simulink model "WW_ST_ESP_ESM_2016a"  (R2017b)
settings: Solver=ode1  StartTime=0.0  StopTime=SIM_time  FixedStep=stepsize  RelTol=1e-3  EnableMultiTasking=on
values from neighbouring files (symbols this model uses):
  A = 2.26    [ST_einspur_parameter.m]
  brems_k_max = 25000    [ST_einspur_parameter.m]
  cw = 0.32    [ST_einspur_parameter.m]
  delta_lr = 0    [ST_einspur_parameter_dynamik.m]    (also in ST_einspur_parameter_sinus.m = 90; ST_einspur_parameter_sprung.m = 90)
  fah_dkv = 0.6    [ST_einspur_parameter_dynamik.m]    (also in ST_einspur_parameter_sinus.m = 0.2; ST_einspur_parameter_sprung.m)
  fzg_Jz = 3489    [ST_einspur_parameter.m]
  fzg_l = 2.758    [ST_einspur_parameter.m]
  fzg_lh = fzg_l-fzg_lv    (= 1.158)    [ST_einspur_parameter.m]
  fzg_lv = 1.6    [ST_einspur_parameter.m]
  fzg_m = 1700    [ST_einspur_parameter.m]
  fzg_s = 1.7    [ST_einspur_parameter.m]
  g = 9.81    [ST_einspur_parameter.m]
  h_sp = 0.56    [ST_einspur_parameter.m]
  i_diff = 3.5    [ST_einspur_parameter.m]
  i_getr = 4.2    [ST_einspur_parameter.m]
  i_lenk = 18    [ST_einspur_parameter.m]
  init_v0 = 5/3.6    (= 1.38888888889)    [ST_einspur_parameter_dynamik.m]    (also in ST_einspur_parameter_sinus.m = 13.8888888889; ST_einspur_parameter_sprung.m = 11.1111111111)
  len_wahl = 1    [ST_einspur_parameter_dynamik.m]    (also in ST_einspur_parameter_sinus.m = 2; ST_einspur_parameter_sprung.m = 3)
  mue_h = 1.0    (= 1)    [ST_einspur_parameter.m]
  mue_v = 1.0    (= 1)    [ST_einspur_parameter.m]
  omega_max = 630    [ST_einspur_parameter.m]
  p_max = 110000    [ST_einspur_parameter.m]
  rad_r = 0.31    [ST_einspur_parameter.m]
  rho = 1.226    [ST_einspur_parameter.m]
  sin_freq = pi/2    (= 1.57079632679)    [ST_einspur_parameter_dynamik.m]    (also in ST_einspur_parameter_sinus.m = 1.0471975512; ST_einspur_parameter_sprung.m)
  step_time = 1    [ST_einspur_parameter_dynamik.m]    (also in ST_einspur_parameter_sinus.m; ST_einspur_parameter_sprung.m = 3)
  sw_ESP = 1    [ST_einspur_parameter_sinus.m]    (also in ST_einspur_parameter_sprung.m)
libraries: simulink x2
(part 2 of 2)

== system WW_ST_ESP_ESM_2016a/Regelsysteme/ESP/Sensorik/Gierratensensor ==
  psi_p : Inport
  Offset : Constant  Value=0.01
  Product : Product  RndMeth=Zero
  Rate Transition : RateTransition
  Rauschamplitude : Constant  Value=0.004
  Sum : Sum  Inputs=+++
  Uniform Random Number : UniformRandomNumber  SampleTime=0.1
  psi_p_mess : Outport
  wires:
  psi_p/1 -> Sum/1
  Product/1 -> Sum/2
  Rauschamplitude/1 -> Product/1
  Rate Transition/1 -> Product/2
  Offset/1 -> Sum/3
  Sum/1 -> psi_p_mess/1
  Uniform Random Number/1 -> Rate Transition/1

== system WW_ST_ESP_ESM_2016a/Regelsysteme/ESP/Sensorik/Schwimmwinkelsensor ==
  beta : Inport
  Offset : Constant  Value=0.01
  Product : Product  RndMeth=Zero
  Rate Transition : RateTransition
  Rauschamplitude : Constant  Value=0.01
  Sum : Sum  Inputs=+++
  Uniform Random Number : UniformRandomNumber  SampleTime=0.1
  beta_mess : Outport
  wires:
  beta/1 -> Sum/1
  Product/1 -> Sum/2
  Rauschamplitude/1 -> Product/1
  Rate Transition/1 -> Product/2
  Offset/1 -> Sum/3
  Sum/1 -> beta_mess/1
  Uniform Random Number/1 -> Rate Transition/1

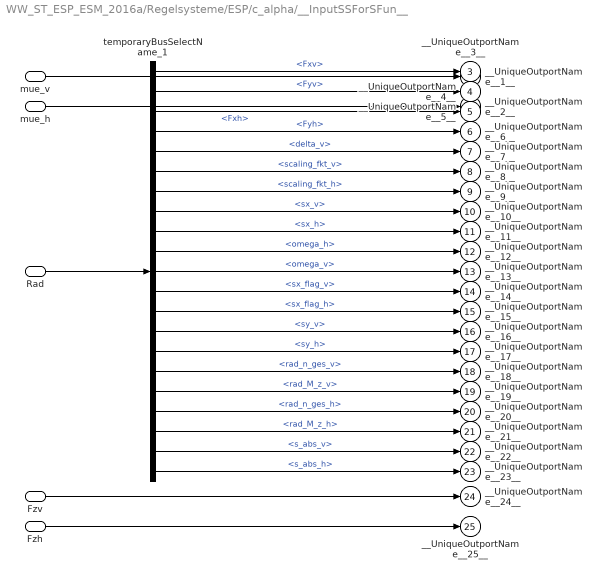
== system WW_ST_ESP_ESM_2016a/Regelsysteme/ESP/c_alpha/__InputSSForSFun__ ==
  mue_v : Inport
  mue_h : Inport  Port=2
  Rad : Inport  Port=3
  Fzv : Inport  Port=4
  Fzh : Inport  Port=5
  temporaryBusSelectName_1 : BusSelector  OutputSignals=Fxv,Fyv,Fxh,Fyh,delta_v,scaling_fkt_v,scaling_fkt_h,sx_v,sx_h,omega_h,omega_v,sx_flag_v,sx_flag_h,sy_v,sy_h,rad_Mz.rad_n_ges_v,rad_Mz.rad_M_z_v,rad_Mz.rad_n_ges_h,rad_Mz.rad_M_z_h,s_abs_v,s_abs_h
  __UniqueOutportName__1__ : Outport
  __UniqueOutportName__2__ : Outport  Port=2
  __UniqueOutportName__3__ : Outport  Port=3
  __UniqueOutportName__4__ : Outport  Port=4
  __UniqueOutportName__5__ : Outport  Port=5
  __UniqueOutportName__6__ : Outport  Port=6
  __UniqueOutportName__7__ : Outport  Port=7
  __UniqueOutportName__8__ : Outport  Port=8
  __UniqueOutportName__9__ : Outport  Port=9
  __UniqueOutportName__10__ : Outport  Port=10
  __UniqueOutportName__11__ : Outport  Port=11
  __UniqueOutportName__12__ : Outport  Port=12
  __UniqueOutportName__13__ : Outport  Port=13
  __UniqueOutportName__14__ : Outport  Port=14
  __UniqueOutportName__15__ : Outport  Port=15
  __UniqueOutportName__16__ : Outport  Port=16
  __UniqueOutportName__17__ : Outport  Port=17
  __UniqueOutportName__18__ : Outport  Port=18
  __UniqueOutportName__19__ : Outport  Port=19
  __UniqueOutportName__20__ : Outport  Port=20
  __UniqueOutportName__21__ : Outport  Port=21
  __UniqueOutportName__22__ : Outport  Port=22
  __UniqueOutportName__23__ : Outport  Port=23
  __UniqueOutportName__24__ : Outport  Port=24
  __UniqueOutportName__25__ : Outport  Port=25
  wires:
  Fzh/1 -> __UniqueOutportName__25__/1
  Fzv/1 -> __UniqueOutportName__24__/1
  temporaryBusSelectName_1/21 -> __UniqueOutportName__23__/1  "<s_abs_h>"
  temporaryBusSelectName_1/20 -> __UniqueOutportName__22__/1  "<s_abs_v>"
  temporaryBusSelectName_1/19 -> __UniqueOutportName__21__/1  "<rad_M_z_h>"
  temporaryBusSelectName_1/18 -> __UniqueOutportName__20__/1  "<rad_n_ges_h>"
  temporaryBusSelectName_1/17 -> __UniqueOutportName__19__/1  "<rad_M_z_v>"
  temporaryBusSelectName_1/16 -> __UniqueOutportName__18__/1  "<rad_n_ges_v>"
  temporaryBusSelectName_1/15 -> __UniqueOutportName__17__/1  "<sy_h>"
  temporaryBusSelectName_1/14 -> __UniqueOutportName__16__/1  "<sy_v>"
  temporaryBusSelectName_1/13 -> __UniqueOutportName__15__/1  "<sx_flag_h>"
  temporaryBusSelectName_1/12 -> __UniqueOutportName__14__/1  "<sx_flag_v>"
  temporaryBusSelectName_1/11 -> __UniqueOutportName__13__/1  "<omega_v>"
  temporaryBusSelectName_1/10 -> __UniqueOutportName__12__/1  "<omega_h>"
  temporaryBusSelectName_1/9 -> __UniqueOutportName__11__/1  "<sx_h>"
  temporaryBusSelectName_1/8 -> __UniqueOutportName__10__/1  "<sx_v>"
  temporaryBusSelectName_1/7 -> __UniqueOutportName__9__/1  "<scaling_fkt_h>"
  temporaryBusSelectName_1/6 -> __UniqueOutportName__8__/1  "<scaling_fkt_v>"
  temporaryBusSelectName_1/5 -> __UniqueOutportName__7__/1  "<delta_v>"
  temporaryBusSelectName_1/4 -> __UniqueOutportName__6__/1  "<Fyh>"
  temporaryBusSelectName_1/3 -> __UniqueOutportName__5__/1  "<Fxh>"
  temporaryBusSelectName_1/2 -> __UniqueOutportName__4__/1  "<Fyv>"
  temporaryBusSelectName_1/1 -> __UniqueOutportName__3__/1  "<Fxv>"
  mue_h/1 -> __UniqueOutportName__2__/1
  mue_v/1 -> __UniqueOutportName__1__/1
  Rad/1 -> temporaryBusSelectName_1/1

== system WW_ST_ESP_ESM_2016a/Regelsysteme/ESP/c_alpha/__OutputSSForSFun__ ==
  __UniqueInportName__1__ : Inport
  __UniqueInportName__2__ : Inport  Port=2
  c_alpha_v : Outport
  c_alpha_h : Outport  Port=2
  wires:
  __UniqueInportName__2__/1 -> c_alpha_h/1
  __UniqueInportName__1__/1 -> c_alpha_v/1

== matlab function WW_ST_ESP_ESM_2016a/Regelsysteme/ESP/Subsystem/D-Anteil ==
  data: psi_p input; y output; v input
function y = fcn(psi_p,v)

% D-Regelparameter von psi_p
if v>=0 & v<=70;
    Kd_psi_p=(-1/70).*v+1;
else if v>70 & v<=100;
        Kd_psi_p =0;
else 
    Kd_psi_p = nan;
    end
end

Kd = 1;

y = Kd.*(Kd_psi_p .* psi_p); % delta_Mz(D)
end

== matlab function WW_ST_ESP_ESM_2016a/Regelsysteme/ESP/Subsystem/Dead Zone ==
  data: u input; y output
function y = fcn(u)

if u > -60 & u < 60;
     y = 0;

else y = u;

    
end

y = u;
end

== matlab function WW_ST_ESP_ESM_2016a/Regelsysteme/ESP/Subsystem/I-Anteil ==
  data: psi_p input; y output; v input
function y = fcn(psi_p,v)

% I-Regelparameter von psi_p
if v>=0 & v<=70;
    Ki_psi_p=(-1/70).*v+1;
else if v>70 & v<=100;
        Ki_psi_p =0;
else 
    Ki_psi_p = nan;
    end
end

Ki = 80;

y = Ki.*(Ki_psi_p .* psi_p);

== matlab function WW_ST_ESP_ESM_2016a/Regelsysteme/ESP/Subsystem/P-Anteil ==
  data: psi_p input; y output; beta input; v input
function y=fcn(psi_p,beta,v)

% P-Regelarameter von psi_p
if v>=0 & v<=70;
    Kp_psi_p=(-1/70).*v+1;
else if v>70 & v<=100;
        Kp_psi_p =0;
else 
    Kp_psi_p = nan;
    end
end

% P-Regelarameter von beta
if  v>=0 & v<=70;
    Kp_beta=(-1/70).*v+1;
else if v>70 & v<=100;
        Kp_beta =0;
else 
    Kp_beta = nan;
    end
end

% beta-Regelparameter

if beta>= pi/30;
    Kp_beta = 1;
else Kp_beta = 0;
end

Kp = 5000;

y = Kp*(Kp_psi_p .* psi_p + Kp_beta .* sign(beta) .* sqrt(abs(beta))); %delta_Mz von P-Anteil
end
